simulink library "rov_design_analysis"  (Simulink 6.0)
settings: Solver=ode45  SolverMode=SingleTasking  StartTime=0.0  StopTime=10.0  RelTol=1e-3
undefined symbols (not defined in the file or in its folder): amp, At, B, Bt, Ct, cycles, D, den, DL, Do, DQ, DQL, freq, frtest, I, L, m, M, Ma, magnitude, MaU, Mt, nmiss, num, phase, rg, sigbuilder_block, slcm, T, W, xb, xg, Xudot, yb, yg, Yvdot, zb, zg, Zwdot
libraries: simulink_extras x32, simulink x27, rov_design_analysis x15, marine_gnc x10, dspmtrx2 x6, dspstat3 x4
(part 4 of 9)

== system rov_design_analysis/ROV Models/ ROMEO ROV (6DoF)   /upper limit (diag)    ==
  note: 7 8 9 10 11 12
  note: 1 2 3 4 5 6
  vel : Inport  Port=1  LatchInput=off
  (zg.W - zb.B)cY.sX : Fcn  Expr=-u[9]*u[3]*u[5]+u[8]*u[2]*u[6]
  (zg.W - zb.B)cY.sX1 : Fcn  Expr=u[9]*u[3]*u[4]-u[7]*u[1]*u[6]
  (zg.W - zb.B)cY.sX2 : Fcn  Expr=-u[8]*u[2]*u[4]+u[7]*u[1]*u[5]
  (zg.W - zb.B)cY.sX3 : Fcn  Expr=-u[9]*u[3]*u[2]+u[8]*u[2]*u[3]-u[12]*u[6]*u[5]+u[11]*u[5]*u[6]
  (zg.W - zb.B)cY.sX4 : Fcn  Expr=u[9]*u[3]*u[1]-u[7]*u[1]*u[3]+u[6]*u[12]*u[4]-u[4]*u[10]*u[6]
  (zg.W - zb.B)cY.sX5 : Fcn  Expr=-u[8]*u[2]*u[1]+u[7]*u[1]*u[2]-u[11]*u[5]*u[4]+u[10]*u[4]*u[5]
  Mux1 : Mux  Inputs=6
  Mux3 : Mux  Inputs=2
  Rg1 : Constant  Value="[Ma(1)  Ma(2)  Ma(3)  Ma(4)  Ma(5)  Ma(6) ]'"
  force : Outport
  wires:
  Mux1/1 -> force/1
  (zg.W - zb.B)cY.sX/1 -> Mux1/1
  (zg.W - zb.B)cY.sX1/1 -> Mux1/2
  (zg.W - zb.B)cY.sX2/1 -> Mux1/3
  (zg.W - zb.B)cY.sX3/1 -> Mux1/4
  (zg.W - zb.B)cY.sX4/1 -> Mux1/5
  (zg.W - zb.B)cY.sX5/1 -> Mux1/6
  vel/1 -> Mux3/1
  Rg1/1 -> Mux3/2
  Mux3/1 -> (zg.W - zb.B)cY.sX/1, (zg.W - zb.B)cY.sX1/1, (zg.W - zb.B)cY.sX4/1, (zg.W - zb.B)cY.sX5/1, (zg.W - zb.B)cY.sX3/1, (zg.W - zb.B)cY.sX2/1

== system rov_design_analysis/ROV Models/ ROMEO ROV (6DoF)   /upper limit (diag)   1 ==
  note: 7 8 9 10 11 12
  note: 1 2 3 4 5 6
  vel : Inport  Port=1  LatchInput=off
  (zg.W - zb.B)cY.sX : Fcn  Expr=-u[9]*u[3]*u[5]+u[8]*u[2]*u[6]
  (zg.W - zb.B)cY.sX1 : Fcn  Expr=u[9]*u[3]*u[4]-u[7]*u[1]*u[6]
  (zg.W - zb.B)cY.sX2 : Fcn  Expr=-u[8]*u[2]*u[4]+u[7]*u[1]*u[5]
  (zg.W - zb.B)cY.sX3 : Fcn  Expr=-u[9]*u[3]*u[2]+u[8]*u[2]*u[3]-u[12]*u[6]*u[5]+u[11]*u[5]*u[6]
  (zg.W - zb.B)cY.sX4 : Fcn  Expr=u[9]*u[3]*u[1]-u[7]*u[1]*u[3]+u[6]*u[12]*u[4]-u[4]*u[10]*u[6]
  (zg.W - zb.B)cY.sX5 : Fcn  Expr=-u[8]*u[2]*u[1]+u[7]*u[1]*u[2]-u[11]*u[5]*u[4]+u[10]*u[4]*u[5]
  Mux1 : Mux  Inputs=6
  Mux3 : Mux  Inputs=2
  Rg1 : Constant  Value="[Ma(1)  Ma(2)  Ma(3)  Ma(4)  Ma(5)  Ma(6) ]'"
  force : Outport
  wires:
  Mux1/1 -> force/1
  (zg.W - zb.B)cY.sX/1 -> Mux1/1
  (zg.W - zb.B)cY.sX1/1 -> Mux1/2
  (zg.W - zb.B)cY.sX2/1 -> Mux1/3
  (zg.W - zb.B)cY.sX3/1 -> Mux1/4
  (zg.W - zb.B)cY.sX4/1 -> Mux1/5
  (zg.W - zb.B)cY.sX5/1 -> Mux1/6
  vel/1 -> Mux3/1
  Rg1/1 -> Mux3/2
  Mux3/1 -> (zg.W - zb.B)cY.sX/1, (zg.W - zb.B)cY.sX1/1, (zg.W - zb.B)cY.sX4/1, (zg.W - zb.B)cY.sX5/1, (zg.W - zb.B)cY.sX3/1, (zg.W - zb.B)cY.sX2/1

== system rov_design_analysis/ROV Models/ ROMEO ROV (6DoF)   /upper limit1 ==
  In : Inport  Port=1  LatchInput=off
  inverse M : Gain  Gain=0  Multiplication=Matrix(K*u)  SaturateOnIntegerOverflow=on
  Out : Outport
  wires:
  inverse M/1 -> Out/1
  In/1 -> inverse M/1

== system rov_design_analysis/ROV Models/1. Nonlinear RRC ROV- unperturbed (6DoF)/Centripetal & Coriolis ==
  vel : Inport  Orientation=up  Port=1  LatchInput=off
  Demux : Demux  Orientation=up  Outputs=2
  Mux : Mux  Inputs=2
  Product{1..5} (5 alike) : Product  SaturateOnIntegerOverflow=on  RndMeth=Zero  InputSameDT=on
  Rg : Constant  Value=rg
  Sum : Sum  SaturateOnIntegerOverflow=on  InputSameDT=on
  Sum1 : Sum  SaturateOnIntegerOverflow=on  InputSameDT=on
  inertia(3x3) : Gain  Gain=I*eye(3)+[Xudot 0 0;0 Yvdot 0;0 0 Zwdot]  Multiplication=Matrix(K*u)  SaturateOnIntegerOverflow=on
  "mass(3x3) " : Gain  Gain=m*eye(3)+[Xudot 0 0;0 Yvdot 0;0 0 Zwdot]  Multiplication=Matrix(K*u)  SaturateOnIntegerOverflow=on
  "mass(3x3)   " : Gain  Gain=m*eye(3)+[Xudot 0 0;0 Yvdot 0;0 0 Zwdot]  Multiplication=Matrix(K*u)  SaturateOnIntegerOverflow=on
  force : Outport  InitialOutput=0
  wires:
  Product1/1 -> Sum/2
  "mass(3x3)   "/1 -> Product2/1
  Product2/1 -> Sum/1
  Rg/1 -> Product3/2, "mass(3x3)   "/1
  Product3/1 -> Product4/2
  Product4/1 -> Sum1/1
  Product5/1 -> Product2/2, Sum1/2
  Sum1/1 -> "mass(3x3) "/1
  Demux/2 -> Product5/1, Product3/1, Product4/1, Product1/1, inertia(3x3)/1
  Demux/1 -> Product5/2
  vel/1 -> Demux/1
  inertia(3x3)/1 -> Product1/2
  "mass(3x3) "/1 -> Mux/1
  Sum/1 -> Mux/2
  Mux/1 -> force/1

== system rov_design_analysis/ROV Models/1. Nonlinear RRC ROV- unperturbed (6DoF)/Hydrodynamic  Damping ==
  vel : Inport  Port=1  LatchInput=off
  Add : Sum  Inputs=--  OutScaling=2^-10
  D linear : Gain  Gain=diag(DL)  SaturateOnIntegerOverflow=on
  D quadratic : Gain  Gain=diag(DQ)  SaturateOnIntegerOverflow=on
  Product : Product  SaturateOnIntegerOverflow=on  RndMeth=Zero  InputSameDT=on
  |u| : Abs  SaturateOnIntegerOverflow=on
  damping force : Outport  InitialOutput=0
  wires:
  Product/1 -> D quadratic/1
  D quadratic/1 -> Add/2
  vel/1 -> |u|/1, Product/1, D linear/1
  |u|/1 -> Product/2
  Add/1 -> damping force/1
  D linear/1 -> Add/1

== system rov_design_analysis/ROV Models/1. Nonlinear RRC ROV- unperturbed (6DoF)/Mass Inertia Matrix ==
  In : Inport  Port=1  LatchInput=off
  inverse M : Gain  Gain=inv(Mt)  Multiplication=Matrix(K*u)  SaturateOnIntegerOverflow=on
  Out : Outport
  wires:
  In/1 -> inverse M/1
  inverse M/1 -> Out/1

== system rov_design_analysis/ROV Models/1. Nonlinear RRC ROV- unperturbed (6DoF)/Model Info ==
  EmptySubsystem : Subsystem

== system rov_design_analysis/ROV Models/1. Nonlinear RRC ROV- unperturbed (6DoF)/More Info ==

== system rov_design_analysis/ROV Models/1. Nonlinear RRC ROV- unperturbed (6DoF)/Restoring Forces ==
  pos : Inport  Port=1  LatchInput=off
  (xg.W-xb.B)cY.cX : Fcn  Expr=(xg*W - xb*B)*cos(u[2])*cos(u[1])
  (zg.W - zb.B)cY.sX : Fcn  Expr=((zg * W - zb * B) * cos(u[2])) * sin(u[1])
  (zg.W - zb.B)sY : Fcn  Expr=(zg*W - zb*B)*sin(u[2])
  -(xg.W-xb.B)cY.sX : Fcn  Expr=-(xg*W - xb*B)*cos(u[2])*sin(u[1])
  -(yg.W-yb.B)cY.cX : Fcn  Expr=-(yg*W - yb*B)*cos(u[2])*cos(u[1])
  -(yg.W-yb.B)sY : Fcn  Expr=-(yg*W - yb*B)*sin(u[2])
  -cY.cX : Fcn  Expr=-cos(u[2])*cos(u[1])
  -cY.sX : Fcn  Expr=-cos(u[2])*sin(u[1])
  Demux : Demux  Outputs=2
  Gain : Gain  Gain=W-B  SaturateOnIntegerOverflow=on
  Mux : Mux  Inputs=3
  Mux1 : Mux
  Sum : Sum  SaturateOnIntegerOverflow=on  InputSameDT=on
  Sum1 : Sum  SaturateOnIntegerOverflow=on  InputSameDT=on
  Sum2 : Sum  SaturateOnIntegerOverflow=on  InputSameDT=on
  Terminator : Terminator
  sY : Fcn  Expr=sin(u[2])
  gravitational force : Outport  InitialOutput=0
  wires:
  pos/1 -> Demux/1
  Demux/1 -> Terminator/1
  Demux/2 -> -cY.cX/1, -cY.sX/1, sY/1, (zg.W - zb.B)cY.sX/1, -(yg.W-yb.B)cY.cX/1, (xg.W-xb.B)cY.cX/1, (zg.W - zb.B)sY/1, -(yg.W-yb.B)sY/1, -(xg.W-xb.B)cY.sX/1
  Mux1/1 -> gravitational force/1
  sY/1 -> Mux/1
  -cY.sX/1 -> Mux/2
  -cY.cX/1 -> Mux/3
  Mux/1 -> Gain/1
  Gain/1 -> Mux1/1
  -(yg.W-yb.B)cY.cX/1 -> Sum/2
  (zg.W - zb.B)cY.sX/1 -> Sum/1
  Sum/1 -> Mux1/2
  (zg.W - zb.B)sY/1 -> Sum1/2
  (xg.W-xb.B)cY.cX/1 -> Sum1/1
  Sum1/1 -> Mux1/3
  -(xg.W-xb.B)cY.sX/1 -> Sum2/2
  -(yg.W-yb.B)sY/1 -> Sum2/1
  Sum2/1 -> Mux1/4

== system rov_design_analysis/ROV Models/1. Nonlinear RRC ROV- unperturbed (6DoF)/show ==

== system rov_design_analysis/ROV Models/JHU ROV (6DoF)   / Load   ==

== system rov_design_analysis/ROV Models/JHU ROV (6DoF)   /Centripetal & Coriolis ==
  vel : Inport  Orientation=up  Port=1  LatchInput=off
  Demux : Demux  Orientation=up  Outputs=2
  Mux : Mux  Inputs=2
  Product{1..5} (5 alike) : Product  SaturateOnIntegerOverflow=on  RndMeth=Zero  InputSameDT=on
  Rg : Constant  Value=rg
  Sum : Sum  SaturateOnIntegerOverflow=on  InputSameDT=on
  Sum1 : Sum  SaturateOnIntegerOverflow=on  InputSameDT=on
  inertia(3x3) : Gain  Gain=I*eye(3)+[0 0 0;0 0 0;0 0 0]  Multiplication=Matrix(K*u)  SaturateOnIntegerOverflow=on
  "mass(3x3) " : Gain  Gain=m*eye(3)+[0 0 0;0 0 0;0 0 0]  Multiplication=Matrix(K*u)  SaturateOnIntegerOverflow=on
  "mass(3x3)   " : Gain  Gain=m*eye(3)+[0 0 0;0 0 0;0 0 0]  Multiplication=Matrix(K*u)  SaturateOnIntegerOverflow=on
  force : Outport  InitialOutput=0
  wires:
  Product1/1 -> Sum/2
  "mass(3x3)   "/1 -> Product2/1
  Product2/1 -> Sum/1
  Rg/1 -> Product3/2, "mass(3x3)   "/1
  Product3/1 -> Product4/2
  Product4/1 -> Sum1/1
  Product5/1 -> Product2/2, Sum1/2
  Sum1/1 -> "mass(3x3) "/1
  Demux/2 -> Product5/1, Product3/1, Product4/1, Product1/1, inertia(3x3)/1
  Demux/1 -> Product5/2
  vel/1 -> Demux/1
  inertia(3x3)/1 -> Product1/2
  "mass(3x3) "/1 -> Mux/1
  Sum/1 -> Mux/2
  Mux/1 -> force/1

== system rov_design_analysis/ROV Models/JHU ROV (6DoF)   /Hydrodynamic  Damping1 ==
  vel : Inport  Port=1  LatchInput=off
  D quadratic : Gain  Gain=-diag(DQ)  SaturateOnIntegerOverflow=on
  Product : Product  SaturateOnIntegerOverflow=on  RndMeth=Zero  InputSameDT=on
  |u| : Abs  SaturateOnIntegerOverflow=on
  damping force : Outport  InitialOutput=0
  wires:
  Product/1 -> D quadratic/1
  vel/1 -> Product/1, |u|/1
  |u|/1 -> Product/2
  D quadratic/1 -> damping force/1

== system rov_design_analysis/ROV Models/JHU ROV (6DoF)   /Hydrodynamic  Damping2 ==
  vel : Inport  Port=1  LatchInput=off
  D quadratic : Gain  Gain=0  SaturateOnIntegerOverflow=on
  damping force : Outport  InitialOutput=0
  wires:
  D quadratic/1 -> damping force/1
  vel/1 -> D quadratic/1

== system rov_design_analysis/ROV Models/JHU ROV (6DoF)   /Mass Inertia Matrix ==
  In : Inport  Port=1  LatchInput=off
  inverse M : Gain  Gain=inv(M-Ma)  Multiplication=Matrix(K*u)  SaturateOnIntegerOverflow=on
  Out : Outport
  wires:
  inverse M/1 -> Out/1
  In/1 -> inverse M/1

== system rov_design_analysis/ROV Models/JHU ROV (6DoF)   /Restoring Forces ==
  pos : Inport  Port=1  LatchInput=off
  (xg.W-xb.B)cY.cX : Fcn  Expr=(xg*W - xb*B)*cos(u[2])*cos(u[1])
  (zg.W - zb.B)cY.sX : Fcn  Expr=((zg * W - zb * B) * cos(u[2])) * sin(u[1])
  -(yg.W-yb.B)sY : Fcn  Expr=0.1197
  -cY.cX : Fcn  Expr=-31.01
  -cY.sX : Fcn  Expr=1.73
  Demux : Demux  Outputs=2
  Mux : Mux  Inputs=3
  Mux1 : Mux
  Terminator : Terminator
  sY : Fcn  Expr=-1.96
  gravitational force : Outport  InitialOutput=0
  wires:
  -(yg.W-yb.B)sY/1 -> Mux1/4
  (xg.W-xb.B)cY.cX/1 -> Mux1/3
  (zg.W - zb.B)cY.sX/1 -> Mux1/2
  Mux/1 -> Mux1/1
  -cY.cX/1 -> Mux/3
  -cY.sX/1 -> Mux/2
  sY/1 -> Mux/1
  Mux1/1 -> gravitational force/1
  Demux/2 -> (zg.W - zb.B)cY.sX/1, (xg.W-xb.B)cY.cX/1, -(yg.W-yb.B)sY/1, sY/1, -cY.sX/1, -cY.cX/1
  Demux/1 -> Terminator/1
  pos/1 -> Demux/1

== system rov_design_analysis/ROV Models/JHU ROV (6DoF)   /pert ==
  In : Inport  Port=1  LatchInput=off
  inp : Inport  Port=2  LatchInput=off
  D linear3 : Gain  Gain=2  SaturateOnIntegerOverflow=on
  Product : Product  RndMeth=Zero
  Sine Wave-pert : Sin  Amplitude=0.1  SampleTime=0
  Sum6 : Sum  Inputs=|++  SaturateOnIntegerOverflow=on  InputSameDT=on
  on/off : Outport
  wires:
  D linear3/1 -> Sum6/1
  Sine Wave-pert/1 -> Product/1
  Product/1 -> Sum6/2
  inp/1 -> Product/2
  In/1 -> D linear3/1
  Sum6/1 -> on/off/1

== system rov_design_analysis/ROV Models/JHU ROV (6DoF)   /pert1 ==
  In : Inport  Port=1  LatchInput=off
  inp : Inport  Port=2  LatchInput=off
  D linear3 : Gain  Gain=2  SaturateOnIntegerOverflow=on
  Product : Product  RndMeth=Zero
  Sine Wave-pert : Sin  Amplitude=0.1  SampleTime=0
  Sum6 : Sum  Inputs=|++  SaturateOnIntegerOverflow=on  InputSameDT=on
  on/off : Outport
  wires:
  D linear3/1 -> Sum6/1
  Sine Wave-pert/1 -> Product/1
  Product/1 -> Sum6/2
  inp/1 -> Product/2
  In/1 -> D linear3/1
  Sum6/1 -> on/off/1

== system rov_design_analysis/ROV Models/JHU ROV (6DoF)   /upper limit (diag) ==
  In : Inport  Port=1  LatchInput=off
  inverse M : Gain  Gain=-diag([21.724-21.1403 51.7013-51.7012 94.3-92.451 4.2176-3.6191 7.1148-2.6427 4.7673-2.3033])  Multiplication=Matrix(K*u)  SaturateOnIntegerOverflow=on
  Out : Outport
  wires:
  inverse M/1 -> Out/1
  In/1 -> inverse M/1

== system rov_design_analysis/ROV Models/JHU ROV (6DoF)   /upper limit (diag)    ==
  note: 7 8 9 10 11 12
  note: 1 2 3 4 5 6
  vel : Inport  Port=1  LatchInput=off
  (zg.W - zb.B)cY.sX : Fcn  Expr=-u[9]*u[3]*u[5]+u[8]*u[2]*u[6]
  (zg.W - zb.B)cY.sX1 : Fcn  Expr=u[9]*u[3]*u[4]-u[7]*u[1]*u[6]
  (zg.W - zb.B)cY.sX2 : Fcn  Expr=-u[8]*u[2]*u[4]+u[7]*u[1]*u[5]
  (zg.W - zb.B)cY.sX3 : Fcn  Expr=-u[9]*u[3]*u[2]+u[8]*u[2]*u[3]-u[12]*u[6]*u[5]+u[11]*u[5]*u[6]
  (zg.W - zb.B)cY.sX4 : Fcn  Expr=u[9]*u[3]*u[1]-u[7]*u[1]*u[3]+u[6]*u[12]*u[4]-u[4]*u[10]*u[6]
  (zg.W - zb.B)cY.sX5 : Fcn  Expr=-u[8]*u[2]*u[1]+u[7]*u[1]*u[2]-u[11]*u[5]*u[4]+u[10]*u[4]*u[5]
  Mux1 : Mux  Inputs=6
  Mux3 : Mux  Inputs=2
  Rg1 : Constant  Value="[Ma(1)  Ma(2)  Ma(3)  Ma(4)  Ma(5)  Ma(6) ]'"
  force : Outport
  wires:
  Mux1/1 -> force/1
  (zg.W - zb.B)cY.sX/1 -> Mux1/1
  (zg.W - zb.B)cY.sX1/1 -> Mux1/2
  (zg.W - zb.B)cY.sX2/1 -> Mux1/3
  (zg.W - zb.B)cY.sX3/1 -> Mux1/4
  (zg.W - zb.B)cY.sX4/1 -> Mux1/5
  (zg.W - zb.B)cY.sX5/1 -> Mux1/6
  vel/1 -> Mux3/1
  Rg1/1 -> Mux3/2
  Mux3/1 -> (zg.W - zb.B)cY.sX/1, (zg.W - zb.B)cY.sX1/1, (zg.W - zb.B)cY.sX4/1, (zg.W - zb.B)cY.sX5/1, (zg.W - zb.B)cY.sX3/1, (zg.W - zb.B)cY.sX2/1

== system rov_design_analysis/ROV Models/JHU ROV (6DoF)   /upper limit (diag)   1 ==
  note: 7 8 9 10 11 12
  note: 1 2 3 4 5 6
  vel : Inport  Port=1  LatchInput=off
  (zg.W - zb.B)cY.sX : Fcn  Expr=-u[9]*u[3]*u[5]+u[8]*u[2]*u[6]
  (zg.W - zb.B)cY.sX1 : Fcn  Expr=u[9]*u[3]*u[4]-u[7]*u[1]*u[6]
  (zg.W - zb.B)cY.sX2 : Fcn  Expr=-u[8]*u[2]*u[4]+u[7]*u[1]*u[5]
  (zg.W - zb.B)cY.sX3 : Fcn  Expr=-u[9]*u[3]*u[2]+u[8]*u[2]*u[3]-u[12]*u[6]*u[5]+u[11]*u[5]*u[6]
  (zg.W - zb.B)cY.sX4 : Fcn  Expr=u[9]*u[3]*u[1]-u[7]*u[1]*u[3]+u[6]*u[12]*u[4]-u[4]*u[10]*u[6]
  (zg.W - zb.B)cY.sX5 : Fcn  Expr=-u[8]*u[2]*u[1]+u[7]*u[1]*u[2]-u[11]*u[5]*u[4]+u[10]*u[4]*u[5]
  Mux1 : Mux  Inputs=6
  Mux3 : Mux  Inputs=2
  Rg1 : Constant  Value="[Ma(1)  Ma(2)  Ma(3)  Ma(4)  Ma(5)  Ma(6) ]'"
  force : Outport
  wires:
  Mux1/1 -> force/1
  (zg.W - zb.B)cY.sX/1 -> Mux1/1
  (zg.W - zb.B)cY.sX1/1 -> Mux1/2
  (zg.W - zb.B)cY.sX2/1 -> Mux1/3
  (zg.W - zb.B)cY.sX3/1 -> Mux1/4
  (zg.W - zb.B)cY.sX4/1 -> Mux1/5
  (zg.W - zb.B)cY.sX5/1 -> Mux1/6
  vel/1 -> Mux3/1
  Rg1/1 -> Mux3/2
  Mux3/1 -> (zg.W - zb.B)cY.sX/1, (zg.W - zb.B)cY.sX1/1, (zg.W - zb.B)cY.sX4/1, (zg.W - zb.B)cY.sX5/1, (zg.W - zb.B)cY.sX3/1, (zg.W - zb.B)cY.sX2/1

== system rov_design_analysis/ROV Models/JHU ROV (6DoF)   /upper limit1 ==
  In : Inport  Port=1  LatchInput=off
  inverse M : Gain  Gain=0  Multiplication=Matrix(K*u)  SaturateOnIntegerOverflow=on
  Out : Outport
  wires:
  inverse M/1 -> Out/1
  In/1 -> inverse M/1

== system rov_design_analysis/ROV Models/Nonlinear RRC ROV - Perturbed (6DoF)   /Centripetal & Coriolis ==
  vel : Inport  Orientation=up  Port=1  LatchInput=off
  Demux : Demux  Orientation=up  Outputs=2
  Mux : Mux  Inputs=2
  Product{1..5} (5 alike) : Product  SaturateOnIntegerOverflow=on  RndMeth=Zero  InputSameDT=on
  Rg : Constant  Value=rg
  Sum : Sum  SaturateOnIntegerOverflow=on  InputSameDT=on
  Sum1 : Sum  SaturateOnIntegerOverflow=on  InputSameDT=on
  inertia(3x3) : Gain  Gain=I*eye(3)+[Xudot 0 0;0 Yvdot 0;0 0 Zwdot]  Multiplication=Matrix(K*u)  SaturateOnIntegerOverflow=on
  "mass(3x3) " : Gain  Gain=m*eye(3)+[Xudot 0 0;0 Yvdot 0;0 0 Zwdot]  Multiplication=Matrix(K*u)  SaturateOnIntegerOverflow=on
  "mass(3x3)   " : Gain  Gain=m*eye(3)+[Xudot 0 0;0 Yvdot 0;0 0 Zwdot]  Multiplication=Matrix(K*u)  SaturateOnIntegerOverflow=on
  force : Outport  InitialOutput=0
  wires:
  Product1/1 -> Sum/2
  "mass(3x3)   "/1 -> Product2/1
  Product2/1 -> Sum/1
  Rg/1 -> Product3/2, "mass(3x3)   "/1
  Product3/1 -> Product4/2
  Product4/1 -> Sum1/1
  Product5/1 -> Product2/2, Sum1/2
  Sum1/1 -> "mass(3x3) "/1
  Demux/2 -> Product5/1, Product3/1, Product4/1, Product1/1, inertia(3x3)/1
  Demux/1 -> Product5/2
  vel/1 -> Demux/1
  inertia(3x3)/1 -> Product1/2
  "mass(3x3) "/1 -> Mux/1
  Sum/1 -> Mux/2
  Mux/1 -> force/1

== system rov_design_analysis/ROV Models/Nonlinear RRC ROV - Perturbed (6DoF)   /Hydrodynamic  Damping ==
  vel : Inport  Port=1  LatchInput=off
  D linear : Gain  Gain=-diag(DQL)  SaturateOnIntegerOverflow=on
  damping force : Outport  InitialOutput=0
  wires:
  vel/1 -> D linear/1
  D linear/1 -> damping force/1

== system rov_design_analysis/ROV Models/Nonlinear RRC ROV - Perturbed (6DoF)   /Hydrodynamic  Damping1 ==
  vel : Inport  Port=1  LatchInput=off
  D quadratic : Gain  Gain=-diag(DQ)  SaturateOnIntegerOverflow=on
  Product : Product  SaturateOnIntegerOverflow=on  RndMeth=Zero  InputSameDT=on
  |u| : Abs  SaturateOnIntegerOverflow=on
  damping force : Outport  InitialOutput=0
  wires:
  Product/1 -> D quadratic/1
  vel/1 -> Product/1, |u|/1
  |u|/1 -> Product/2
  D quadratic/1 -> damping force/1

== system rov_design_analysis/ROV Models/Nonlinear RRC ROV - Perturbed (6DoF)   /Hydrodynamic  Damping2 ==
  vel : Inport  Port=1  LatchInput=off
  D quadratic : Gain  Gain=0  SaturateOnIntegerOverflow=on
  damping force : Outport  InitialOutput=0
  wires:
  D quadratic/1 -> damping force/1
  vel/1 -> D quadratic/1

== system rov_design_analysis/ROV Models/Nonlinear RRC ROV - Perturbed (6DoF)   /Mass Inertia Matrix ==
  In : Inport  Port=1  LatchInput=off
  inverse M : Gain  Gain=inv(M-Ma)  Multiplication=Matrix(K*u)  SaturateOnIntegerOverflow=on
  Out : Outport
  wires:
  inverse M/1 -> Out/1
  In/1 -> inverse M/1

== system rov_design_analysis/ROV Models/Nonlinear RRC ROV - Perturbed (6DoF)   /Restoring Forces ==
  pos : Inport  Port=1  LatchInput=off
  (xg.W-xb.B)cY.cX : Fcn  Expr=(xg*W - xb*B)*cos(u[2])*cos(u[1])
  (zg.W - zb.B)cY.sX : Fcn  Expr=((zg * W - zb * B) * cos(u[2])) * sin(u[1])
  (zg.W - zb.B)sY : Fcn  Expr=(zg*W - zb*B)*sin(u[2])
  -(xg.W-xb.B)cY.sX : Fcn  Expr=-(xg*W - xb*B)*cos(u[2])*sin(u[1])
  -(yg.W-yb.B)cY.cX : Fcn  Expr=-(yg*W - yb*B)*cos(u[2])*cos(u[1])
  -(yg.W-yb.B)sY : Fcn  Expr=-(yg*W - yb*B)*sin(u[2])
  -cY.cX : Fcn  Expr=-cos(u[2])*cos(u[1])
  -cY.sX : Fcn  Expr=-cos(u[2])*sin(u[1])
  Demux : Demux  Outputs=2
  Gain : Gain  Gain=W-B  SaturateOnIntegerOverflow=on
  Mux : Mux  Inputs=3
  Mux1 : Mux
  Sum : Sum  SaturateOnIntegerOverflow=on  InputSameDT=on
  Sum1 : Sum  SaturateOnIntegerOverflow=on  InputSameDT=on
  Sum2 : Sum  SaturateOnIntegerOverflow=on  InputSameDT=on
  Terminator : Terminator
  sY : Fcn  Expr=sin(u[2])
  gravitational force : Outport  InitialOutput=0
  wires:
  Sum2/1 -> Mux1/4
  -(yg.W-yb.B)sY/1 -> Sum2/1
  -(xg.W-xb.B)cY.sX/1 -> Sum2/2
  Sum1/1 -> Mux1/3
  (xg.W-xb.B)cY.cX/1 -> Sum1/1
  (zg.W - zb.B)sY/1 -> Sum1/2
  Sum/1 -> Mux1/2
  (zg.W - zb.B)cY.sX/1 -> Sum/1
  -(yg.W-yb.B)cY.cX/1 -> Sum/2
  Gain/1 -> Mux1/1
  Mux/1 -> Gain/1
  -cY.cX/1 -> Mux/3
  -cY.sX/1 -> Mux/2
  sY/1 -> Mux/1
  Mux1/1 -> gravitational force/1
  Demux/2 -> -(xg.W-xb.B)cY.sX/1, -(yg.W-yb.B)sY/1, (zg.W - zb.B)sY/1, (xg.W-xb.B)cY.cX/1, -(yg.W-yb.B)cY.cX/1, (zg.W - zb.B)cY.sX/1, sY/1, -cY.sX/1, -cY.cX/1
  Demux/1 -> Terminator/1
  pos/1 -> Demux/1

== system rov_design_analysis/ROV Models/Nonlinear RRC ROV - Perturbed (6DoF)   /lower limit (diag) ==
  In : Inport  Port=1  LatchInput=off
  inverse M : Gain  Gain=-diag([21.1403-21.0981 51.7012-51.0026 92.451-91.837 3.6191-3.576 2.6427-2.7687 2.3033-2.3493])  Multiplication=Matrix(K*u)  SaturateOnIntegerOverflow=on
  Out : Outport
  wires:
  inverse M/1 -> Out/1
  In/1 -> inverse M/1

== system rov_design_analysis/ROV Models/Nonlinear RRC ROV - Perturbed (6DoF)   /pert ==
  In : Inport  Port=1  LatchInput=off
  inp : Inport  Port=2  LatchInput=off
  D linear3 : Gain  Gain=2  SaturateOnIntegerOverflow=on
  Product : Product  RndMeth=Zero
  Sine Wave-pert : Sin  Amplitude=0.1  SampleTime=0
  Sum6 : Sum  Inputs=|++  SaturateOnIntegerOverflow=on  InputSameDT=on
  on/off : Outport
  wires:
  D linear3/1 -> Sum6/1
  Sine Wave-pert/1 -> Product/1
  Product/1 -> Sum6/2
  inp/1 -> Product/2
  In/1 -> D linear3/1
  Sum6/1 -> on/off/1

== system rov_design_analysis/ROV Models/Nonlinear RRC ROV - Perturbed (6DoF)   /pert1 ==
  In : Inport  Port=1  LatchInput=off
  inp : Inport  Port=2  LatchInput=off
  D linear3 : Gain  Gain=2  SaturateOnIntegerOverflow=on
  Product : Product  RndMeth=Zero
  Sine Wave-pert : Sin  Amplitude=0.1  SampleTime=0
  Sum6 : Sum  Inputs=|++  SaturateOnIntegerOverflow=on  InputSameDT=on
  on/off : Outport
  wires:
  D linear3/1 -> Sum6/1
  Sine Wave-pert/1 -> Product/1
  Product/1 -> Sum6/2
  inp/1 -> Product/2
  In/1 -> D linear3/1
  Sum6/1 -> on/off/1

== system rov_design_analysis/ROV Models/Nonlinear RRC ROV - Perturbed (6DoF)   /pert2 ==
  In : Inport  Port=1  LatchInput=off
  inp : Inport  Port=2  LatchInput=off
  D linear3 : Gain  Gain=2  SaturateOnIntegerOverflow=on
  Product : Product  RndMeth=Zero
  Sine Wave-pert : Sin  Amplitude=0.1  SampleTime=0
  Sum6 : Sum  Inputs=|++  SaturateOnIntegerOverflow=on  InputSameDT=on
  on/off : Outport
  wires:
  D linear3/1 -> Sum6/1
  Sine Wave-pert/1 -> Product/1
  Product/1 -> Sum6/2
  inp/1 -> Product/2
  In/1 -> D linear3/1
  Sum6/1 -> on/off/1

== system rov_design_analysis/ROV Models/Nonlinear RRC ROV - Perturbed (6DoF)   /upper limit (diag) ==
  In : Inport  Port=1  LatchInput=off
  inverse M : Gain  Gain=-diag([21.724-21.1403 51.7013-51.7012 94.3-92.451 4.2176-3.6191 7.1148-2.6427 4.7673-2.3033])  Multiplication=Matrix(K*u)  SaturateOnIntegerOverflow=on
  Out : Outport
  wires:
  inverse M/1 -> Out/1
  In/1 -> inverse M/1

== system rov_design_analysis/ROV Models/Nonlinear RRC ROV - Perturbed (6DoF)   /upper limit (diag)    ==
  note: 7 8 9 10 11 12
  note: 1 2 3 4 5 6
  vel : Inport  Port=1  LatchInput=off
  (zg.W - zb.B)cY.sX : Fcn  Expr=-u[9]*u[3]*u[5]+u[8]*u[2]*u[6]
  (zg.W - zb.B)cY.sX1 : Fcn  Expr=u[9]*u[3]*u[4]-u[7]*u[1]*u[6]
  (zg.W - zb.B)cY.sX2 : Fcn  Expr=-u[8]*u[2]*u[4]+u[7]*u[1]*u[5]
  (zg.W - zb.B)cY.sX3 : Fcn  Expr=-u[9]*u[3]*u[2]+u[8]*u[2]*u[3]-u[12]*u[6]*u[5]+u[11]*u[5]*u[6]
  (zg.W - zb.B)cY.sX4 : Fcn  Expr=u[9]*u[3]*u[1]-u[7]*u[1]*u[3]+u[6]*u[12]*u[4]-u[4]*u[10]*u[6]
  (zg.W - zb.B)cY.sX5 : Fcn  Expr=-u[8]*u[2]*u[1]+u[7]*u[1]*u[2]-u[11]*u[5]*u[4]+u[10]*u[4]*u[5]
  Mux1 : Mux  Inputs=6
  Mux3 : Mux  Inputs=2
  Rg1 : Constant  Value="[MaU(1)  MaU(2)  MaU(3)  MaU(4)  MaU(5)  MaU(6) ]'"
  force : Outport
  wires:
  Mux1/1 -> force/1
  (zg.W - zb.B)cY.sX/1 -> Mux1/1
  (zg.W - zb.B)cY.sX1/1 -> Mux1/2
  (zg.W - zb.B)cY.sX2/1 -> Mux1/3
  (zg.W - zb.B)cY.sX3/1 -> Mux1/4
  (zg.W - zb.B)cY.sX4/1 -> Mux1/5
  (zg.W - zb.B)cY.sX5/1 -> Mux1/6
  vel/1 -> Mux3/1
  Rg1/1 -> Mux3/2
  Mux3/1 -> (zg.W - zb.B)cY.sX/1, (zg.W - zb.B)cY.sX1/1, (zg.W - zb.B)cY.sX4/1, (zg.W - zb.B)cY.sX5/1, (zg.W - zb.B)cY.sX3/1, (zg.W - zb.B)cY.sX2/1

== system rov_design_analysis/ROV Models/Nonlinear RRC ROV - Perturbed (6DoF)   /upper limit (diag)   1 ==
  note: 7 8 9 10 11 12
  note: 1 2 3 4 5 6
  vel : Inport  Port=1  LatchInput=off
  (zg.W - zb.B)cY.sX : Fcn  Expr=-u[9]*u[3]*u[5]+u[8]*u[2]*u[6]
  (zg.W - zb.B)cY.sX1 : Fcn  Expr=u[9]*u[3]*u[4]-u[7]*u[1]*u[6]
  (zg.W - zb.B)cY.sX2 : Fcn  Expr=-u[8]*u[2]*u[4]+u[7]*u[1]*u[5]
  (zg.W - zb.B)cY.sX3 : Fcn  Expr=-u[9]*u[3]*u[2]+u[8]*u[2]*u[3]-u[12]*u[6]*u[5]+u[11]*u[5]*u[6]
  (zg.W - zb.B)cY.sX4 : Fcn  Expr=u[9]*u[3]*u[1]-u[7]*u[1]*u[3]+u[6]*u[12]*u[4]-u[4]*u[10]*u[6]
  (zg.W - zb.B)cY.sX5 : Fcn  Expr=-u[8]*u[2]*u[1]+u[7]*u[1]*u[2]-u[11]*u[5]*u[4]+u[10]*u[4]*u[5]
  Mux1 : Mux  Inputs=6
  Mux3 : Mux  Inputs=2
  Rg1 : Constant  Value="[Ma(1)  Ma(2)  Ma(3)  Ma(4)  Ma(5)  Ma(6) ]'"
  force : Outport
  wires:
  Mux1/1 -> force/1
  (zg.W - zb.B)cY.sX/1 -> Mux1/1
  (zg.W - zb.B)cY.sX1/1 -> Mux1/2
  (zg.W - zb.B)cY.sX2/1 -> Mux1/3
  (zg.W - zb.B)cY.sX3/1 -> Mux1/4
  (zg.W - zb.B)cY.sX4/1 -> Mux1/5
  (zg.W - zb.B)cY.sX5/1 -> Mux1/6
  vel/1 -> Mux3/1
  Rg1/1 -> Mux3/2
  Mux3/1 -> (zg.W - zb.B)cY.sX/1, (zg.W - zb.B)cY.sX1/1, (zg.W - zb.B)cY.sX4/1, (zg.W - zb.B)cY.sX5/1, (zg.W - zb.B)cY.sX3/1, (zg.W - zb.B)cY.sX2/1

== system rov_design_analysis/ROV Models/Nonlinear RRC ROV - Perturbed (6DoF)   /upper limit1 ==
  In : Inport  Port=1  LatchInput=off
  inverse M : Gain  Gain=0  Multiplication=Matrix(K*u)  SaturateOnIntegerOverflow=on
  Out : Outport
  wires:
  inverse M/1 -> Out/1
  In/1 -> inverse M/1

== system rov_design_analysis/ROV Models/Thruster Configuration Matrix of RRC ROV  (6X4)/row vector 1 ==
  T11 : Inport  Port=1  LatchInput=off
  T12 : Inport  Port=2  LatchInput=off
  T13 : Inport  Port=3  LatchInput=off
  T14 : Inport  Port=4  LatchInput=off
  Thruster column vector (1) : simulink/Math Operations/Matrix Concatenation  numInports=4  catMethod=Horizontal
  row 1 : Outport
  wires:
  Thruster column vector (1)/1 -> row 1/1
  T11/1 -> Thruster column vector (1)/1
  T12/1 -> Thruster column vector (1)/2
  T13/1 -> Thruster column vector (1)/3
  T14/1 -> Thruster column vector (1)/4

== system rov_design_analysis/ROV Models/Thruster Configuration Matrix of RRC ROV  (6X4)/row vector 2 ==
  T21 : Inport  Port=1  LatchInput=off
  T22 : Inport  Port=2  LatchInput=off
  T23 : Inport  Port=3  LatchInput=off
  T24 : Inport  Port=4  LatchInput=off
  "   " : Trigonometry
  "   1" : Trigonometry
  Thruster column vector (2) : simulink/Math Operations/Matrix Concatenation  numInports=4  catMethod=Horizontal
  sign : Gain
  sign1 : Gain  Gain=-1
  row 2 : Outport
  wires:
  Thruster column vector (2)/1 -> row 2/1
  T21/1 -> Thruster column vector (2)/1
  T22/1 -> Thruster column vector (2)/2
  "   "/1 -> Thruster column vector (2)/3
  T24/1 -> sign1/1
  sign1/1 -> "   1"/1
  "   1"/1 -> Thruster column vector (2)/4
  T23/1 -> sign/1
  sign/1 -> "   "/1

== system rov_design_analysis/ROV Models/Thruster Configuration Matrix of RRC ROV  (6X4)/row vector 3 ==
  T31 : Inport  Port=1  LatchInput=off
  T32 : Inport  Port=2  LatchInput=off
  T33 : Inport  Port=3  LatchInput=off
  T34 : Inport  Port=4  LatchInput=off
  "   " : Trigonometry  Operator=cos
  "   1" : Trigonometry  Operator=cos
  Thruster column vector (1) : simulink/Math Operations/Matrix Concatenation  numInports=4  catMethod=Horizontal
  sign : Gain
  sign1 : Gain
  row 3 : Outport
  wires:
  Thruster column vector (1)/1 -> row 3/1
  T31/1 -> Thruster column vector (1)/1
  T32/1 -> Thruster column vector (1)/2
  sign1/1 -> "   1"/1
  sign/1 -> "   "/1
  "   "/1 -> Thruster column vector (1)/3
  "   1"/1 -> Thruster column vector (1)/4
  T33/1 -> sign/1
  T34/1 -> sign1/1

== system rov_design_analysis/ROV Models/Thruster Configuration Matrix of RRC ROV  (6X4)/row vector 4 ==
  T41 : Inport  Port=1  LatchInput=off
  T42 : Inport  Port=2  LatchInput=off
  T43 : Inport  Port=3  LatchInput=off
  T44 : Inport  Port=4  LatchInput=off
  Gain : Gain
  Thruster column vector (2) : simulink/Math Operations/Matrix Concatenation  numInports=4  catMethod=Horizontal
  sign : Gain  Gain=-1
  row 4 : Outport
  wires:
  Thruster column vector (2)/1 -> row 4/1
  T41/1 -> Thruster column vector (2)/1
  T42/1 -> Thruster column vector (2)/2
  T43/1 -> sign/1
  sign/1 -> Thruster column vector (2)/3
  T44/1 -> Gain/1
  Gain/1 -> Thruster column vector (2)/4

== system rov_design_analysis/ROV Models/Thruster Configuration Matrix of RRC ROV  (6X4)/row vector 5 ==
  T51 : Inport  Port=1  LatchInput=off
  T52 : Inport  Port=2  LatchInput=off
  T53 : Inport  Port=3  LatchInput=off
  T54 : Inport  Port=4  LatchInput=off
  Gain : Gain  Gain=-1
  Gain1 : Gain  Gain=-1
  Gain2 : Gain  Gain=-1
  Product : Product  RndMeth=Zero
  Thruster column vector (1) : simulink/Math Operations/Matrix Concatenation  numInports=4  catMethod=Horizontal
  Trigonometric Function : Trigonometry  Operator=cos
  row 5 : Outport
  wires:
  Thruster column vector (1)/1 -> row 5/1
  T51/1 -> Gain/1
  Gain/1 -> Thruster column vector (1)/1
  T52/1 -> Gain1/1
  Gain1/1 -> Thruster column vector (1)/2
  T54/1 -> Product/2
  T53/1 -> Trigonometric Function/1
  Trigonometric Function/1 -> Product/1
  Product/1 -> Gain2/1
  Gain2/1 -> Thruster column vector (1)/3, Thruster column vector (1)/4

== system rov_design_analysis/ROV Models/Thruster Configuration Matrix of RRC ROV  (6X4)/row vector 6 ==
  T61 : Inport  Port=1  LatchInput=off
  T62 : Inport  Port=2  LatchInput=off
  T63 : Inport  Port=3  LatchInput=off
  T64 : Inport  Port=4  LatchInput=off
  Gain : Gain
  Gain1 : Gain  Gain=-1
  Gain2 : Gain
  Gain3 : Gain  Gain=-1
  Product : Product  RndMeth=Zero
  Thruster column vector (1) : simulink/Math Operations/Matrix Concatenation  numInports=4  catMethod=Horizontal
  Trigonometric Function : Trigonometry
  row 6 : Outport
  wires:
  Thruster column vector (1)/1 -> row 6/1
  T61/1 -> Gain/1
  Gain/1 -> Thruster column vector (1)/1
  T62/1 -> Gain1/1
  Gain1/1 -> Thruster column vector (1)/2
  T64/1 -> Product/2
  T63/1 -> Trigonometric Function/1
  Trigonometric Function/1 -> Product/1
  Product/1 -> Gain2/1, Gain3/1
  Gain2/1 -> Thruster column vector (1)/3
  Gain3/1 -> Thruster column vector (1)/4

== system rov_design_analysis/ROV Controller / Hamiltonian  Interconnection-Damping Assignment  - 2 DoF/Model Info ==
  EmptySubsystem : Subsystem

== system rov_design_analysis/ROV Controller / Multi-controller selection -  4 DoF/controller 1 ==
  PID : Inport  Port=1  LatchInput=off
  Demux1 : Demux
  Mux2 : Mux
  PID Controller{1..3,6} (4 alike) : simulink_extras/Additional Linear/PID Controller  P=11  I=10  D=1
  "Output " : Outport
  wires:
  Demux1/1 -> PID Controller1/1
  Demux1/2 -> PID Controller2/1
  Demux1/3 -> PID Controller3/1
  PID Controller1/1 -> Mux2/1
  PID Controller2/1 -> Mux2/2
  PID Controller3/1 -> Mux2/3
  PID Controller6/1 -> Mux2/4
  PID/1 -> Demux1/1
  Mux2/1 -> "Output "/1
  Demux1/4 -> PID Controller6/1

== system rov_design_analysis/ROV Controller / Multi-controller selection -  4 DoF/controller 2 ==
  PI : Inport  Port=1  LatchInput=off
  Demux1 : Demux
  Mux2 : Mux
  PD Controller{1..4} (4 alike) : simulink_extras/Additional Linear/PID Controller  P=11  I=0  D=1
  "Output " : Outport
  wires:
  Demux1/4 -> PD Controller4/1
  Mux2/1 -> "Output "/1
  PI/1 -> Demux1/1
  PD Controller4/1 -> Mux2/4
  PD Controller3/1 -> Mux2/3
  PD Controller2/1 -> Mux2/2
  PD Controller1/1 -> Mux2/1
  Demux1/3 -> PD Controller3/1
  Demux1/2 -> PD Controller2/1
  Demux1/1 -> PD Controller1/1

== system rov_design_analysis/ROV Controller / Multi-controller selection -  4 DoF/controller 3 ==
  PID : Inport  Port=1  LatchInput=off
  Demux1 : Demux
  Mux2 : Mux
  PI Controller1 : simulink_extras/Additional Linear/PID Controller  P=11  I=10  D=0
  PI Controller2 : simulink_extras/Additional Linear/PID Controller  P=11  I=10  D=0
  PI Controller4 : simulink_extras/Additional Linear/PID Controller  P=11  I=10  D=0
  PID Controller3 : simulink_extras/Additional Linear/PID Controller  P=11  I=10  D=0
  "Output " : Outport
  wires:
  Demux1/4 -> PI Controller4/1
  Mux2/1 -> "Output "/1
  PID/1 -> Demux1/1
  PI Controller4/1 -> Mux2/4
  PID Controller3/1 -> Mux2/3
  PI Controller2/1 -> Mux2/2
  PI Controller1/1 -> Mux2/1
  Demux1/3 -> PID Controller3/1
  Demux1/2 -> PI Controller2/1
  Demux1/1 -> PI Controller1/1

== system rov_design_analysis/ROV Controller / Open-loop ROV - 6 DoF/Model Info ==
  EmptySubsystem : Subsystem

== system rov_design_analysis/ROV Controller /Adaptive PD  Cascaded  Controller - 6 DoF/Body-fixed to Earth_fixed Transformation1 ==
  Input earth Velocity : Inport  Port=1  LatchInput=off
  Demux : Demux  Outputs=2
  Demux1 : Demux  Outputs=2
  Intregrator2 : Integrator
  Mux1 : Mux  Inputs=2
  Terminator : Terminator
  Transformation matrix R : Subsystem
      mask Display: disp('Transformation R')
  Transformation matrix T : Subsystem
      mask Display: disp('Transformation T')
  Output body velocities : Outport  InitialOutput=0
  wires:
  Intregrator2/1 -> Demux1/1
  Mux1/1 -> Output body velocities/1, Intregrator2/1
  Input earth Velocity/1 -> Demux/1
  Demux1/1 -> Terminator/1
  Transformation matrix T/1(translational earth velocity) -> Mux1/1
  Transformation matrix R/1(angular earth velocity) -> Mux1/2
  Demux1/2 -> Transformation matrix R/2(angular position), Transformation matrix T/2(angular position)
  Demux/1 -> Transformation matrix T/1(translational body velocity)
  Demux/2 -> Transformation matrix R/1(angular body  velocity)

== system rov_design_analysis/ROV Controller /Adaptive PD  Cascaded  Controller - 6 DoF/Body-fixed to Earth_fixed Transformation3 ==
  Input earth Velocity : Inport  Port=1  LatchInput=off
  Demux : Demux  Outputs=2
  Demux1 : Demux  Outputs=2
  Intregrator2 : Integrator
  Mux1 : Mux  Inputs=2
  Terminator : Terminator
  Transformation matrix R : Subsystem
      mask Display: disp('Transformation R')
  Transformation matrix T : Subsystem
      mask Display: disp('Transformation T')
  Output body velocities : Outport  InitialOutput=0
  wires:
  Demux/2 -> Transformation matrix R/1(angular body  velocity)
  Demux/1 -> Transformation matrix T/1(translational body velocity)
  Demux1/2 -> Transformation matrix T/2(angular position), Transformation matrix R/2(angular position)
  Transformation matrix R/1(angular earth velocity) -> Mux1/2
  Transformation matrix T/1(translational earth velocity) -> Mux1/1
  Demux1/1 -> Terminator/1
  Input earth Velocity/1 -> Demux/1
  Mux1/1 -> Intregrator2/1, Output body velocities/1
  Intregrator2/1 -> Demux1/1

== system rov_design_analysis/ROV Controller /Adaptive PD  Cascaded  Controller - 6 DoF/Pseudo Inverse (n X n) ==
  In1 : Inport  Port=1  LatchInput=off
  Gain : Gain  Gain=pinv(T)  Multiplication=Matrix(K*u)
  Out1 : Outport
  wires:
  Gain/1 -> Out1/1
  In1/1 -> Gain/1

== system rov_design_analysis/ROV Controller /Adaptive PD  Cascaded  Controller - 6 DoF/Subsystem2 ==
  note: 2nd order
      | dynamic thruster model
  "Input " : Inport  Port=1  LatchInput=off
  Demux1 : Demux
  Mux2 : Mux
  SubSystem11 : Subsystem
  SubSystem12 : Subsystem
  SubSystem5 : Subsystem
  SubSystem6 : Subsystem
  "Output " : Outport
  wires:
  Demux1/1 -> SubSystem12/1(volt)
  SubSystem12/1(thrust) -> Mux2/1
  Demux1/2 -> SubSystem5/1(volt)
  SubSystem5/1(thrust) -> Mux2/2
  SubSystem6/1(thrust) -> Mux2/3
  Demux1/3 -> SubSystem6/1(volt)
  Demux1/4 -> SubSystem11/1(volt)
  SubSystem11/1(thrust) -> Mux2/4
  Mux2/1 -> "Output "/1
  "Input "/1 -> Demux1/1

== system rov_design_analysis/ROV Controller /Adaptive PD  Cascaded  Controller - 6 DoF/kd ==
  body vel : Inport  Port=1  LatchInput=off
  Demux : Demux  Outputs=6
  Mux : Mux  Inputs=6
  kd1 : Gain  Gain=22  SaturateOnIntegerOverflow=on
  kd2 : Gain  Gain=27  SaturateOnIntegerOverflow=on
  kd3 : Gain  Gain=3  SaturateOnIntegerOverflow=on
  kd4 : Gain  Gain=2.6  SaturateOnIntegerOverflow=on
  kd5 : Gain  Gain=3  SaturateOnIntegerOverflow=on
  kd6 : Gain  Gain=10  SaturateOnIntegerOverflow=on
  kd : Outport
  wires:
  Mux/1 -> kd/1
  body vel/1 -> Demux/1
  Demux/1 -> kd1/1
  Demux/2 -> kd2/1
  Demux/3 -> kd3/1
  Demux/4 -> kd4/1
  Demux/5 -> kd5/1
  Demux/6 -> kd6/1
  kd1/1 -> Mux/1
  kd2/1 -> Mux/2
  kd3/1 -> Mux/3
  kd4/1 -> Mux/4
  kd5/1 -> Mux/5
  kd6/1 -> Mux/6

== system rov_design_analysis/ROV Controller /Adaptive PD  Cascaded  Controller - 6 DoF/kp  ==
  body vel : Inport  Port=1  LatchInput=off
  Demux : Demux  Outputs=6
  Mux : Mux  Inputs=6
  kp1 : Gain  Gain=111  SaturateOnIntegerOverflow=on
  kp2 : Gain  Gain=200  SaturateOnIntegerOverflow=on
  kp3 : Gain  Gain=120  SaturateOnIntegerOverflow=on
  kp4 : Gain  Gain=4  SaturateOnIntegerOverflow=on
  kp5 : Gain  Gain=2  SaturateOnIntegerOverflow=on
  kp6 : Gain  Gain=10  SaturateOnIntegerOverflow=on
  kp : Outport
  wires:
  Mux/1 -> kp/1
  body vel/1 -> Demux/1
  Demux/1 -> kp1/1
  Demux/2 -> kp2/1
  Demux/3 -> kp3/1
  Demux/4 -> kp4/1
  Demux/5 -> kp5/1
  Demux/6 -> kp6/1
  kp1/1 -> Mux/1
  kp2/1 -> Mux/2
  kp3/1 -> Mux/3
  kp4/1 -> Mux/4
  kp5/1 -> Mux/5
  kp6/1 -> Mux/6

== system rov_design_analysis/ROV Controller /Adaptive PD  Cascaded  Controller - 6 DoF/pipe tracking profile  (Manual) ==
  Mux : Mux  Inputs=6
  phi : Step  Time=0  After=0  SampleTime=0
  theta : Step  Time=0  After=-50  SampleTime=0
  x : Step  Time=0  After=0  SampleTime=0
  y : Step  Time=0  After=0  SampleTime=0
  yaw : Step  Time=0  After=-1.57  SampleTime=0
  z : Step  Time=0  After=-50  SampleTime=0
  manual : Outport
  wires:
  Mux/1 -> manual/1
  z/1 -> Mux/3
  y/1 -> Mux/2
  x/1 -> Mux/1
  yaw/1 -> Mux/6
  phi/1 -> Mux/4
  theta/1 -> Mux/5

== system rov_design_analysis/ROV Controller /Hybrid Control- one DoF/Body-fixed to Earth_fixed Transformation1 ==
  Input earth Velocity : Inport  Port=1  LatchInput=off
  Demux : Demux  Outputs=2
  Demux1 : Demux  Outputs=2
  Intregrator2 : Integrator
  Mux1 : Mux  Inputs=2
  Terminator : Terminator
  Transformation matrix R : Subsystem
      mask Display: disp('Transformation R')
  Transformation matrix T : Subsystem
      mask Display: disp('Transformation T')
  Output body velocities : Outport  InitialOutput=0
  wires:
  Demux/2 -> Transformation matrix R/1(angular body  velocity)
  Demux/1 -> Transformation matrix T/1(translational body velocity)
  Demux1/2 -> Transformation matrix T/2(angular position), Transformation matrix R/2(angular position)
  Transformation matrix R/1(angular earth velocity) -> Mux1/2
  Transformation matrix T/1(translational earth velocity) -> Mux1/1
  Demux1/1 -> Terminator/1
  Input earth Velocity/1 -> Demux/1
  Mux1/1 -> Intregrator2/1, Output body velocities/1
  Intregrator2/1 -> Demux1/1

== system rov_design_analysis/ROV Controller /Hybrid Control- one DoF/Body-fixed to Earth_fixed Transformation3 ==
  Input earth Velocity : Inport  Port=1  LatchInput=off
  Demux : Demux  Outputs=2
  Demux1 : Demux  Outputs=2
  Intregrator2 : Integrator
  Mux1 : Mux  Inputs=2
  Terminator : Terminator
  Transformation matrix R : Subsystem
      mask Display: disp('Transformation R')
  Transformation matrix T : Subsystem
      mask Display: disp('Transformation T')
  Output body velocities : Outport  InitialOutput=0
  wires:
  Intregrator2/1 -> Demux1/1
  Mux1/1 -> Output body velocities/1, Intregrator2/1
  Input earth Velocity/1 -> Demux/1
  Demux1/1 -> Terminator/1
  Transformation matrix T/1(translational earth velocity) -> Mux1/1
  Transformation matrix R/1(angular earth velocity) -> Mux1/2
  Demux1/2 -> Transformation matrix R/2(angular position), Transformation matrix T/2(angular position)
  Demux/1 -> Transformation matrix T/1(translational body velocity)
  Demux/2 -> Transformation matrix R/1(angular body  velocity)

== system rov_design_analysis/ROV Controller /Hybrid Control- one DoF/Pseudo Inverse (n X n) ==
  In1 : Inport  Port=1  LatchInput=off
  Gain : Gain  Gain=pinv(T)  Multiplication=Matrix(K*u)
  Out1 : Outport
  wires:
  In1/1 -> Gain/1
  Gain/1 -> Out1/1

== system rov_design_analysis/ROV Controller /Hybrid Control- one DoF/Subsystem2 ==
  note: 2nd order
      | dynamic thruster model
  "Input " : Inport  Port=1  LatchInput=off
  Demux1 : Demux
  Mux2 : Mux
  SubSystem11 : Subsystem
  SubSystem12 : Subsystem
  SubSystem5 : Subsystem
  SubSystem6 : Subsystem
  "Output " : Outport
  wires:
  "Input "/1 -> Demux1/1
  Mux2/1 -> "Output "/1
  SubSystem11/1(thrust) -> Mux2/4
  Demux1/4 -> SubSystem11/1(volt)
  Demux1/3 -> SubSystem6/1(volt)
  SubSystem6/1(thrust) -> Mux2/3
  SubSystem5/1(thrust) -> Mux2/2
  Demux1/2 -> SubSystem5/1(volt)
  SubSystem12/1(thrust) -> Mux2/1
  Demux1/1 -> SubSystem12/1(volt)

== system rov_design_analysis/ROV Controller /Hybrid Control- one DoF/kd ==
  body vel : Inport  Port=1  LatchInput=off
  Demux : Demux  Outputs=6
  Mux : Mux  Inputs=6
  kd1 : Gain  Gain=22  SaturateOnIntegerOverflow=on
  kd2 : Gain  Gain=27  SaturateOnIntegerOverflow=on
  kd3 : Gain  Gain=3  SaturateOnIntegerOverflow=on
  kd4 : Gain  Gain=2.6  SaturateOnIntegerOverflow=on
  kd5 : Gain  Gain=3  SaturateOnIntegerOverflow=on
  kd6 : Gain  Gain=10  SaturateOnIntegerOverflow=on
  kd : Outport
  wires:
  kd6/1 -> Mux/6
  kd5/1 -> Mux/5
  kd4/1 -> Mux/4
  kd3/1 -> Mux/3
  kd2/1 -> Mux/2
  kd1/1 -> Mux/1
  Demux/6 -> kd6/1
  Demux/5 -> kd5/1
  Demux/4 -> kd4/1
  Demux/3 -> kd3/1
  Demux/2 -> kd2/1
  Demux/1 -> kd1/1
  body vel/1 -> Demux/1
  Mux/1 -> kd/1

== system rov_design_analysis/ROV Controller /Hybrid Control- one DoF/kp  ==
  body vel : Inport  Port=1  LatchInput=off
  Demux : Demux  Outputs=6
  Mux : Mux  Inputs=6
  kp1 : Gain  Gain=111  SaturateOnIntegerOverflow=on
  kp2 : Gain  Gain=200  SaturateOnIntegerOverflow=on
  kp3 : Gain  Gain=120  SaturateOnIntegerOverflow=on
  kp4 : Gain  Gain=4  SaturateOnIntegerOverflow=on
  kp5 : Gain  Gain=2  SaturateOnIntegerOverflow=on
  kp6 : Gain  Gain=10  SaturateOnIntegerOverflow=on
  kp : Outport
  wires:
  kp6/1 -> Mux/6
  kp5/1 -> Mux/5
  kp4/1 -> Mux/4
  kp3/1 -> Mux/3
  kp2/1 -> Mux/2
  kp1/1 -> Mux/1
  Demux/6 -> kp6/1
  Demux/5 -> kp5/1
  Demux/4 -> kp4/1
  Demux/3 -> kp3/1
  Demux/2 -> kp2/1
  Demux/1 -> kp1/1
  body vel/1 -> Demux/1
  Mux/1 -> kp/1

== system rov_design_analysis/ROV Controller /Hybrid Control- one DoF/pipe tracking profile  (Manual) ==
  Mux : Mux  Inputs=6
  phi : Step  Time=0  After=0  SampleTime=0
  theta : Step  Time=0  After=-50  SampleTime=0
  x : Step  Time=0  After=0  SampleTime=0
  y : Step  Time=0  After=0  SampleTime=0
  yaw : Step  Time=0  After=-1.57  SampleTime=0
  z : Step  Time=0  After=-50  SampleTime=0
  manual : Outport
  wires:
  theta/1 -> Mux/5
  phi/1 -> Mux/4
  yaw/1 -> Mux/6
  x/1 -> Mux/1
  y/1 -> Mux/2
  z/1 -> Mux/3
  Mux/1 -> manual/1

== system rov_design_analysis/ROV Controller /Nonlinear-Based PD  Cascaded  Controller - 6 DoF/Body-fixed to Earth_fixed Transformation1 ==
  Input earth Velocity : Inport  Port=1  LatchInput=off
  Demux : Demux  Outputs=2
  Demux1 : Demux  Outputs=2
  Intregrator2 : Integrator
  Mux1 : Mux  Inputs=2
  Terminator : Terminator
  Transformation matrix R : Subsystem
      mask Display: disp('Transformation R')
  Transformation matrix T : Subsystem
      mask Display: disp('Transformation T')
  Output body velocities : Outport  InitialOutput=0
  wires:
  Demux/2 -> Transformation matrix R/1(angular body  velocity)
  Demux/1 -> Transformation matrix T/1(translational body velocity)
  Demux1/2 -> Transformation matrix T/2(angular position), Transformation matrix R/2(angular position)
  Transformation matrix R/1(angular earth velocity) -> Mux1/2
  Transformation matrix T/1(translational earth velocity) -> Mux1/1
  Demux1/1 -> Terminator/1
  Input earth Velocity/1 -> Demux/1
  Mux1/1 -> Intregrator2/1, Output body velocities/1
  Intregrator2/1 -> Demux1/1

== system rov_design_analysis/ROV Controller /Nonlinear-Based PD  Cascaded  Controller - 6 DoF/Body-fixed to Earth_fixed Transformation3 ==
  Input earth Velocity : Inport  Port=1  LatchInput=off
  Demux : Demux  Outputs=2
  Demux1 : Demux  Outputs=2
  Intregrator2 : Integrator
  Mux1 : Mux  Inputs=2
  Terminator : Terminator
  Transformation matrix R : Subsystem
      mask Display: disp('Transformation R')
  Transformation matrix T : Subsystem
      mask Display: disp('Transformation T')
  Output body velocities : Outport  InitialOutput=0
  wires:
  Intregrator2/1 -> Demux1/1
  Mux1/1 -> Output body velocities/1, Intregrator2/1
  Input earth Velocity/1 -> Demux/1
  Demux1/1 -> Terminator/1
  Transformation matrix T/1(translational earth velocity) -> Mux1/1
  Transformation matrix R/1(angular earth velocity) -> Mux1/2
  Demux1/2 -> Transformation matrix R/2(angular position), Transformation matrix T/2(angular position)
  Demux/1 -> Transformation matrix T/1(translational body velocity)
  Demux/2 -> Transformation matrix R/1(angular body  velocity)

== system rov_design_analysis/ROV Controller /Nonlinear-Based PD  Cascaded  Controller - 6 DoF/Pseudo Inverse (n X n) ==
  In1 : Inport  Port=1  LatchInput=off
  Gain : Gain  Gain=pinv(T)  Multiplication=Matrix(K*u)
  Out1 : Outport
  wires:
  In1/1 -> Gain/1
  Gain/1 -> Out1/1

== system rov_design_analysis/ROV Controller /Nonlinear-Based PD  Cascaded  Controller - 6 DoF/Subsystem2 ==
  note: 2nd order
      | dynamic thruster model
  "Input " : Inport  Port=1  LatchInput=off
  Demux1 : Demux
  Mux2 : Mux
  SubSystem11 : Subsystem
  SubSystem12 : Subsystem
  SubSystem5 : Subsystem
  SubSystem6 : Subsystem
  "Output " : Outport
  wires:
  "Input "/1 -> Demux1/1
  Mux2/1 -> "Output "/1
  SubSystem11/1(thrust) -> Mux2/4
  Demux1/4 -> SubSystem11/1(volt)
  Demux1/3 -> SubSystem6/1(volt)
  SubSystem6/1(thrust) -> Mux2/3
  SubSystem5/1(thrust) -> Mux2/2
  Demux1/2 -> SubSystem5/1(volt)
  SubSystem12/1(thrust) -> Mux2/1
  Demux1/1 -> SubSystem12/1(volt)

== system rov_design_analysis/ROV Controller /Nonlinear-Based PD  Cascaded  Controller - 6 DoF/kd ==
  body vel : Inport  Port=1  LatchInput=off
  Demux : Demux  Outputs=6
  Mux : Mux  Inputs=6
  kd1 : Gain  Gain=22  SaturateOnIntegerOverflow=on
  kd2 : Gain  Gain=27  SaturateOnIntegerOverflow=on
  kd3 : Gain  Gain=3  SaturateOnIntegerOverflow=on
  kd4 : Gain  Gain=2.6  SaturateOnIntegerOverflow=on
  kd5 : Gain  Gain=3  SaturateOnIntegerOverflow=on
  kd6 : Gain  Gain=10  SaturateOnIntegerOverflow=on
  kd : Outport
  wires:
  kd6/1 -> Mux/6
  kd5/1 -> Mux/5
  kd4/1 -> Mux/4
  kd3/1 -> Mux/3
  kd2/1 -> Mux/2
  kd1/1 -> Mux/1
  Demux/6 -> kd6/1
  Demux/5 -> kd5/1
  Demux/4 -> kd4/1
  Demux/3 -> kd3/1
  Demux/2 -> kd2/1
  Demux/1 -> kd1/1
  body vel/1 -> Demux/1
  Mux/1 -> kd/1

== system rov_design_analysis/ROV Controller /Nonlinear-Based PD  Cascaded  Controller - 6 DoF/kp  ==
  body vel : Inport  Port=1  LatchInput=off
  Demux : Demux  Outputs=6
  Mux : Mux  Inputs=6
  kp1 : Gain  Gain=111  SaturateOnIntegerOverflow=on
  kp2 : Gain  Gain=200  SaturateOnIntegerOverflow=on
  kp3 : Gain  Gain=120  SaturateOnIntegerOverflow=on
  kp4 : Gain  Gain=4  SaturateOnIntegerOverflow=on
  kp5 : Gain  Gain=2  SaturateOnIntegerOverflow=on
  kp6 : Gain  Gain=10  SaturateOnIntegerOverflow=on
  kp : Outport
  wires:
  kp6/1 -> Mux/6
  kp5/1 -> Mux/5
  kp4/1 -> Mux/4
  kp3/1 -> Mux/3
  kp2/1 -> Mux/2
  kp1/1 -> Mux/1
  Demux/6 -> kp6/1
  Demux/5 -> kp5/1
  Demux/4 -> kp4/1
  Demux/3 -> kp3/1
  Demux/2 -> kp2/1
  Demux/1 -> kp1/1
  body vel/1 -> Demux/1
  Mux/1 -> kp/1

== system rov_design_analysis/ROV Controller /Nonlinear-Based PD  Cascaded  Controller - 6 DoF/pipe tracking profile  (Manual) ==
  Mux : Mux  Inputs=6
  phi : Step  Time=0  After=0  SampleTime=0
  theta : Step  Time=0  After=-50  SampleTime=0
  x : Step  Time=0  After=0  SampleTime=0
  y : Step  Time=0  After=0  SampleTime=0
  yaw : Step  Time=0  After=-1.57  SampleTime=0
  z : Step  Time=0  After=-50  SampleTime=0
  manual : Outport
  wires:
  theta/1 -> Mux/5
  phi/1 -> Mux/4
  yaw/1 -> Mux/6
  x/1 -> Mux/1
  y/1 -> Mux/2
  z/1 -> Mux/3
  Mux/1 -> manual/1

== system rov_design_analysis/ROV Controller /Nonlinear-Sliding-Mode Cascaded  Controller - 6 DoF/Body-fixed to Earth_fixed Transformation1 ==
  Input earth Velocity : Inport  Port=1  LatchInput=off
  Demux : Demux  Outputs=2
  Demux1 : Demux  Outputs=2
  Intregrator2 : Integrator
  Mux1 : Mux  Inputs=2
  Terminator : Terminator
  Transformation matrix R : Subsystem
      mask Display: disp('Transformation R')
  Transformation matrix T : Subsystem
      mask Display: disp('Transformation T')
  Output body velocities : Outport  InitialOutput=0
  wires:
  Intregrator2/1 -> Demux1/1
  Mux1/1 -> Output body velocities/1, Intregrator2/1
  Input earth Velocity/1 -> Demux/1
  Demux1/1 -> Terminator/1
  Transformation matrix T/1(translational earth velocity) -> Mux1/1
  Transformation matrix R/1(angular earth velocity) -> Mux1/2
  Demux1/2 -> Transformation matrix R/2(angular position), Transformation matrix T/2(angular position)
  Demux/1 -> Transformation matrix T/1(translational body velocity)
  Demux/2 -> Transformation matrix R/1(angular body  velocity)

== system rov_design_analysis/ROV Controller /Nonlinear-Sliding-Mode Cascaded  Controller - 6 DoF/Body-fixed to Earth_fixed Transformation3 ==
  Input earth Velocity : Inport  Port=1  LatchInput=off
  Demux : Demux  Outputs=2
  Demux1 : Demux  Outputs=2
  Intregrator2 : Integrator
  Mux1 : Mux  Inputs=2
  Terminator : Terminator
  Transformation matrix R : Subsystem
      mask Display: disp('Transformation R')
  Transformation matrix T : Subsystem
      mask Display: disp('Transformation T')
  Output body velocities : Outport  InitialOutput=0
  wires:
  Demux/2 -> Transformation matrix R/1(angular body  velocity)
  Demux/1 -> Transformation matrix T/1(translational body velocity)
  Demux1/2 -> Transformation matrix T/2(angular position), Transformation matrix R/2(angular position)
  Transformation matrix R/1(angular earth velocity) -> Mux1/2
  Transformation matrix T/1(translational earth velocity) -> Mux1/1
  Demux1/1 -> Terminator/1
  Input earth Velocity/1 -> Demux/1
  Mux1/1 -> Intregrator2/1, Output body velocities/1
  Intregrator2/1 -> Demux1/1

== system rov_design_analysis/ROV Controller /Nonlinear-Sliding-Mode Cascaded  Controller - 6 DoF/Pseudo Inverse (n X n) ==
  In1 : Inport  Port=1  LatchInput=off
  Gain : Gain  Gain=pinv(T)  Multiplication=Matrix(K*u)
  Out1 : Outport
  wires:
  Gain/1 -> Out1/1
  In1/1 -> Gain/1
